simulink model "noise_model_simulink_spectrum_sb_19a"  (R2019a)
settings: Solver=VariableStepAuto  StartTime=0.0  StopTime=60  RelTol=1e-3
libraries: dspsrcs4 x1
settings Model: Creator=Carolina  LastModifiedBy=sbuccelli

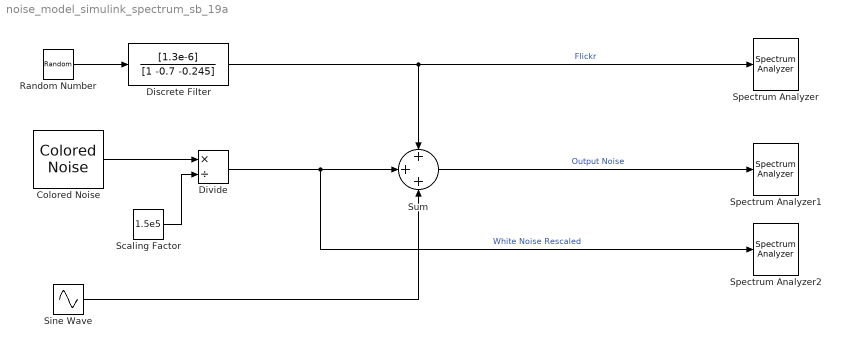
== system noise_model_simulink_spectrum_sb_19a ==
  Colored Noise : dspsrcs4/Colored Noise  Color=white  InverseFrequencyPower=1  NumChannels=1  OutputDataType=double  SamplesPerFrame=1  SampleTime=1/24414  RandomStream=mt19937ar with seed  Seed=67  SimulateUsing=Interpreted execution
      settings: SourceProductName=DSP System Toolbox  SourceProductBaseCode=DS
  Discrete Filter : DiscreteFilter  Numerator=[1.3e-6]  Denominator=[1 -0.7 -0.245]
  Divide : Product  Inputs=*/
  Random Number : RandomNumber  SampleTime=1/24414
  Scaling Factor : Constant  Value=1.5e5
  Sine Wave : Sin  Amplitude=0.6e-6  Frequency=314.16  SampleTime=1/24414
  Spectrum Analyzer : SpectrumAnalyzer
  Spectrum Analyzer1 : SpectrumAnalyzer
  Spectrum Analyzer2 : SpectrumAnalyzer
  Sum : Sum  Inputs=+++
  wires:
  Sine Wave/1 -> Sum/3
  Sum/1 -> Spectrum Analyzer1/1  "Output Noise"
  Random Number/1 -> Discrete Filter/1
  Colored Noise/1 -> Divide/1
  Divide/1 -> Spectrum Analyzer2/1, Sum/2  "White Noise Rescaled"
  Scaling Factor/1 -> Divide/2
  Discrete Filter/1 -> Sum/1, Spectrum Analyzer/1  "Flickr"
